simulink model "HSF_ESC"  (R2018a)
settings: Solver=VariableStepAuto  StartTime=0.0  StopTime=5  RelTol=1e-3
libraries: simulink x1
settings Model: Creator=research  LastModifiedBy=Abdullah Bin Masood

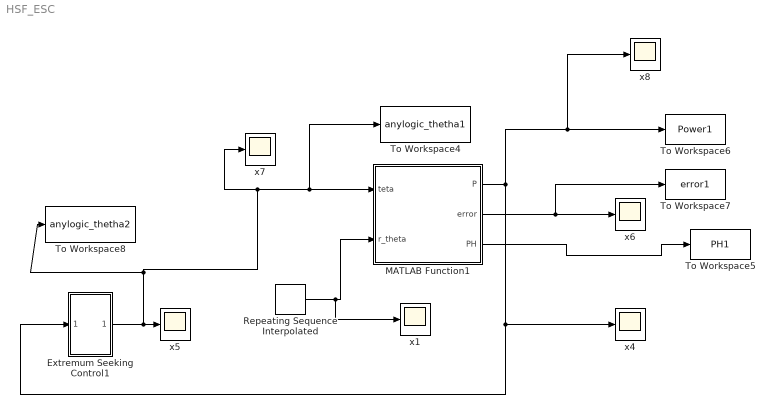
== system HSF_ESC ==
  Extremum Seeking Control1 : Subsystem
  MATLAB Function1 : MATLAB Function  TreatAsAtomicUnit=on
  Repeating Sequence Interpolated : simulink/Sources/Repeating Sequence Interpolated  OutValues="[60\t58\t56\t54\t52\t50\t48\t46\t44\t42\t40].'"  TimeValues=[0 : 10].'  LookUpMeth=Interpolation-Use End Values  tsamp=0.001  OutMin=[]  OutMax=[]  OutDataTypeStr=double  OutputDataTypeScalingMode=double  OutDataType=fixdt(0,8)  OutScaling=2^-10
  To Workspace4 : ToWorkspace  VariableName=anylogic_thetha1  SaveFormat=Timeseries  SampleTime=-1
  To Workspace5 : ToWorkspace  VariableName=PH1  SaveFormat=Timeseries  SampleTime=-1
  To Workspace6 : ToWorkspace  VariableName=Power1  SaveFormat=Timeseries  SampleTime=-1
  To Workspace7 : ToWorkspace  VariableName=error1  SaveFormat=Timeseries  SampleTime=-1
  To Workspace8 : ToWorkspace  VariableName=anylogic_thetha2  SaveFormat=Timeseries  SampleTime=-1
  x{1,4..8} (6 alike) : Scope
  wires:
  MATLAB Function1/1(P) -> x8/1, To Workspace6/1, Extremum Seeking Control1/1(In1), x4/1
  MATLAB Function1/2(error) -> To Workspace7/1, x6/1
  MATLAB Function1/3(PH) -> To Workspace5/1
  Extremum Seeking Control1/1(Out1) -> x7/1, To Workspace4/1, MATLAB Function1/1(teta), To Workspace8/1, x5/1
  Repeating Sequence Interpolated/1 -> x1/1, MATLAB Function1/2(r_theta)

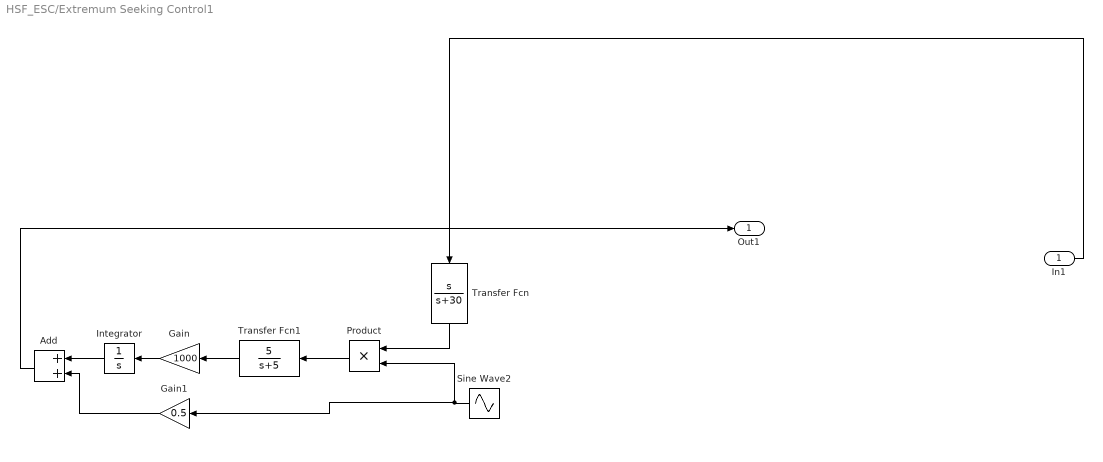
== system HSF_ESC/Extremum Seeking Control1 ==
  In1 : Inport
  Add : Sum
  Gain : Gain  Gain=1000
  Gain1 : Gain  Gain=0.5
  Integrator : Integrator  InitialCondition=55
  Product : Product  RndMeth=Zero
  Sine Wave2 : Sin  Frequency=100  SampleTime=0
  Transfer Fcn : TransferFcn  Numerator=[1 0]  Denominator=[1 30]
  Transfer Fcn1 : TransferFcn  Numerator=[5]  Denominator=[1 5]
  Out1 : Outport
  wires:
  In1/1 -> Transfer Fcn/1
  Add/1 -> Out1/1
  Gain/1 -> Integrator/1
  Transfer Fcn/1 -> Product/1
  Product/1 -> Transfer Fcn1/1
  Integrator/1 -> Add/1
  Gain1/1 -> Add/2
  Transfer Fcn1/1 -> Gain/1
  Sine Wave2/1 -> Gain1/1, Product/2

== matlab function HSF_ESC/MATLAB Function1 ==
  data: teta input; P output; error output; PH output; r_theta input
function [P, error, PH] = HSF(teta, r_theta)
%#codegen


bit=2;
c=299792458;
f=8.65e9;
lambda=c/f;
k = 2*pi/lambda;        
fi=80;
%teta=40;
n=bit;
E=2*pi/2^n*linspace(0,2^n-1,2^n); %whats this?
        phiR=(fi-180)*pi/180;
        thetaR=(teta)*pi/180;
        du=lambda/4;
        DN=6*lambda;  %whats this? Number of unit cells in a row or column
        DM=DN;
        dsx = du*2*pi*cos(phiR)*sin(thetaR)/lambda;   %incident angle is zero so other term is zero
        dsy = du*2*pi*sin(phiR)*sin(thetaR)/lambda;   %incident angle is zero so other term is zero
        M=round(DM/du);
        N=round(DN/du);
        B=zeros(M,N);
        C=B;
        D=C;
        for i=1:M
            for j=1:N
                B(i,j) =((i*dsx) + (j*dsy));       
                C(i,j) = B(i,j);

                while B(i,j)>=2*pi
                    B(i,j)=B(i,j)-2*pi;
                end
                while B(i,j)<0
                    B(i,j)=B(i,j)+2*pi;
                end
                D(i,j)=B(i,j);
                [q, p]=min(abs(E-abs(B(i,j))));
                B(i,j)=E(p);
                if B(i,j)==2*pi
                B(i,j)=0;
                end
            end
        end
       dG=du;Ps=179;Ts=181;
        phi=linspace(-1,180,Ps);
        theta=linspace(-1,91,Ts);
        new = zeros(181, 179);
        F = complex(new, 0); %what is this
        PH = zeros(M,N);
        for a=1:M
            for b=1:N
                PH(a,b)=B(a,b);
                phase = exp(-1j*(PH(a,b) + k*dG*(a-0.5).*sin(theta*pi/180)'*cos(phi*pi/180) + k*dG*(b-0.5).*sin(theta*pi/180)'*sin(phi*pi/180)));
                
                F = F + phase;
                
            end
        end
        
        test= abs(F);
        test_max = max(max(test));
        test_norm = test/test_max;
       % check = max(max(test_norm))
        r_phi=80, 
       % r_theta = 50;
        
       
        
        
        
        [m1,n1]= (min(abs(theta - r_theta))); %what is r_theta
        [m2,n2]= (min(abs(phi - r_phi)));  
        P = test_norm(n1, n2);
        error= teta - r_theta;
        
%         surf(PH)
%         view(0,90)
%         xlim([1 M])
%         ylim([1 N])        
%     
%         figure,
%         surf(phi,theta,abs(F).^2)
%         view(0,90)
%         xlim([0 180])
%         ylim([0 90])
